simulink model "model_sys"  (R2021a)
settings: Solver=VariableStepAuto  StartTime=0.0  StopTime=100  RelTol=1e-3
values from neighbouring files (symbols this model uses):
  A = [-0.3149 235.8928 0 ... (first row only)    [main.m]    (also in rscale.m = a)
  B = [-5.5079 ... (first row only)    [main.m]    (also in rscale.m = b)
  C = [0 0 1]    [main.m]    (also in rscale.m = c)
  K = lqr(A,B,Q,R)    [main.m]    (also in rscale.m = k)
  N = rscale(A,B,C,D,K)    [main.m]    (also in rscale.m = inv([A,B;C,D])*Z')
undefined symbols (not defined in the file or in its folder): Kf
libraries: simulink x2
settings Model: Creator=artof  LastModifiedBy=artof
settings SolverCC: AlgebraicLoopSolver=TrustRegion
settings DebuggingCC: SFMachineParentedDataDiag=warning

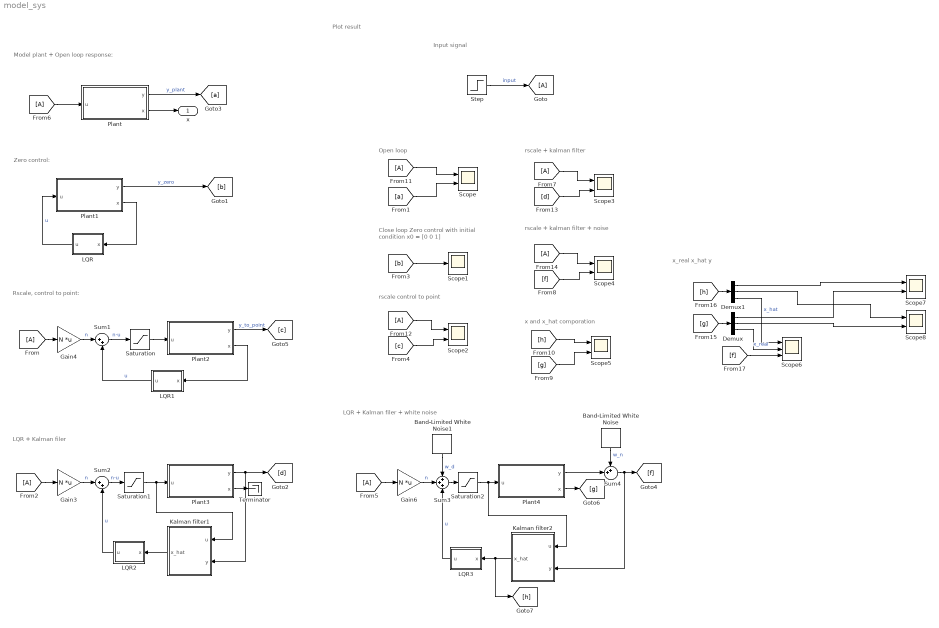
== system model_sys ==
  note: x_real x_hat y
  note: Plot result
  note: Open loop
  note: Input signal
  note: Rscale, control to point:
  note: Zero control:
  note: Model plant + Open loop response:
  note: LQR + Kalman filer
  note: LQR + Kalman filer + white noise
  note: Close loop Zero control with
      | initial condition x0 = [0 0 1]
  note: rscale control to point
  note: rscale + kalman filter
  note: rscale + kalman filter + noise
  note: x and x_hat comporation
  Band-Limited White Noise : simulink/Sources/Band-Limited White Noise  Cov=[0.01]  Ts=0.1  seed=0
  Band-Limited White Noise1 : simulink/Sources/Band-Limited White Noise  Cov=[0.001]  Ts=0.1  seed=0
  Demux : Demux  Outputs=3
  Demux1 : Demux  Outputs=3
  Gain3 : Gain  Gain=N  Multiplication=Matrix(K*u)
  Gain4 : Gain  Gain=N  Multiplication=Matrix(K*u)
  Gain6 : Gain  Gain=N  Multiplication=Matrix(K*u)
  Kalman filter1 : Subsystem
  Kalman filter2 : Subsystem
  LQR : Subsystem
  LQR1 : Subsystem
  LQR2 : Subsystem
  LQR3 : Subsystem
  Plant : Subsystem
  Plant1 : Subsystem
  Plant2 : Subsystem
  Plant3 : Subsystem
  Plant4 : Subsystem
  Saturation : Saturate  UpperLimit=1  LowerLimit=-1
  Saturation1 : Saturate  UpperLimit=1  LowerLimit=-1
  Saturation2 : Saturate  UpperLimit=1  LowerLimit=-1
  Scope{,2..5,7..8} (7 alike) : Scope  NumInputPorts=2
  Scope1 : Scope
  Scope6 : Scope  NumInputPorts=3
  Step : Step  SampleTime=0
  Sum1 : Sum  Inputs=|++
  Sum2 : Sum  Inputs=|++
  Sum3 : Sum  Inputs=+++
  Sum4 : Sum  Inputs=++|
  Terminator : Terminator
  x : Outport
  wires:
  Gain4/1 -> Sum1/1  "n"
  [A] -> Plant/1(u)
  Plant/1(y) -> [a]  "y_plant"
  LQR/1(u) -> Plant1/1(u)  "u"
  Plant/2(x) -> x/1
  Plant1/1(y) -> [b]  "y_zero"
  Plant1/2(x) -> LQR/1(x)
  Plant2/2(x) -> LQR1/1(x)
  LQR1/1(u) -> Sum1/2  "u"
  Gain3/1 -> Sum2/1  "n"
  LQR2/1(u) -> Sum2/2  "u"
  Plant3/1(y) -> [d], Kalman filter1/2(y)
  Sum2/1 -> Saturation1/1  "n-u"
  Gain6/1 -> Sum3/2  "n"
  LQR3/1(u) -> Sum3/3  "u"
  Band-Limited White Noise1/1 -> Sum3/1  "w_d"
  Step/1 -> [A]  "input"
  [a] -> Scope/2
  [A] -> Gain4/1
  Plant2/1(y) -> [c]  "y_to_point"
  [A] -> Gain3/1
  [b] -> Scope1/1
  [c] -> Scope2/2
  [A] -> Gain6/1
  Plant3/2(x) -> Terminator/1
  Kalman filter1/1(x_hat) -> LQR2/1(x)
  Kalman filter2/1(x_hat) -> [h], LQR3/1(x)
  Plant4/1(y) -> Sum4/2
  Plant4/2(x) -> [g]
  Band-Limited White Noise/1 -> Sum4/1  "w_n"
  Sum4/1 -> Kalman filter2/2(y), [f]
  [h] -> Scope5/1
  [g] -> Scope5/2
  [A] -> Scope/1
  [A] -> Scope2/1
  [A] -> Scope3/1
  [d] -> Scope3/2
  [A] -> Scope4/1
  [f] -> Scope4/2
  [g] -> Demux/1
  [h] -> Demux1/1
  Demux1/3 -> Scope6/1  "x_hat"
  Demux/3 -> Scope6/2  "x_real"
  [f] -> Scope6/3
  Sum1/1 -> Saturation/1  "n-u"
  Saturation/1 -> Plant2/1(u)
  Saturation1/1 -> Kalman filter1/1(u), Plant3/1(u)
  Sum3/1 -> Saturation2/1
  Saturation2/1 -> Kalman filter2/1(u), Plant4/1(u)
  Demux1/1 -> Scope7/1
  Demux/1 -> Scope7/2
  Demux1/2 -> Scope8/1
  Demux/2 -> Scope8/2

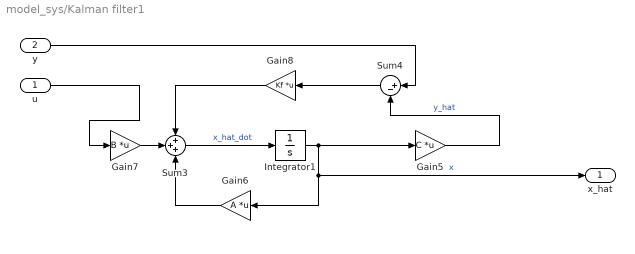
== system model_sys/Kalman filter1 ==
  u : Inport
  y : Inport  Port=2
  Gain5 : Gain  Gain=C  Multiplication=Matrix(K*u)
  Gain6 : Gain  Gain=A  Multiplication=Matrix(K*u)
  Gain7 : Gain  Gain=B  Multiplication=Matrix(K*u)
  Gain8 : Gain  Gain=Kf  Multiplication=Matrix(K*u)
  Integrator1 : Integrator
  Sum3 : Sum  Inputs=+++
  Sum4 : Sum  Inputs=|+-
  x_hat : Outport
  wires:
  Gain5/1 -> Sum4/2  "y_hat"
  Gain6/1 -> Sum3/3
  Gain7/1 -> Sum3/2
  Sum4/1 -> Gain8/1
  Sum3/1 -> Integrator1/1  "x_hat_dot"
  y/1 -> Sum4/1
  Integrator1/1 -> Gain5/1, x_hat/1, Gain6/1  "x"
  Gain8/1 -> Sum3/1
  u/1 -> Gain7/1

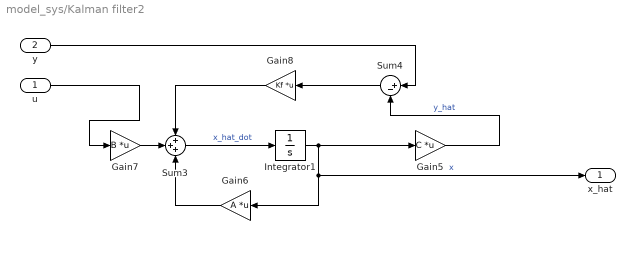
== system model_sys/Kalman filter2 ==
  u : Inport
  y : Inport  Port=2
  Gain5 : Gain  Gain=C  Multiplication=Matrix(K*u)
  Gain6 : Gain  Gain=A  Multiplication=Matrix(K*u)
  Gain7 : Gain  Gain=B  Multiplication=Matrix(K*u)
  Gain8 : Gain  Gain=Kf  Multiplication=Matrix(K*u)
  Integrator1 : Integrator
  Sum3 : Sum  Inputs=+++
  Sum4 : Sum  Inputs=|+-
  x_hat : Outport
  wires:
  Gain5/1 -> Sum4/2  "y_hat"
  Gain6/1 -> Sum3/3
  Gain7/1 -> Sum3/2
  Sum4/1 -> Gain8/1
  Sum3/1 -> Integrator1/1  "x_hat_dot"
  y/1 -> Sum4/1
  Integrator1/1 -> Gain5/1, x_hat/1, Gain6/1  "x"
  Gain8/1 -> Sum3/1
  u/1 -> Gain7/1

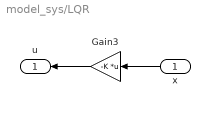
== system model_sys/LQR ==
  x : Inport
  Gain3 : Gain  Gain=-K  Multiplication=Matrix(K*u)
  u : Outport
  wires:
  x/1 -> Gain3/1
  Gain3/1 -> u/1

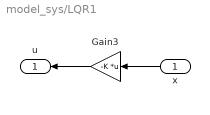
== system model_sys/LQR1 ==
  x : Inport
  Gain3 : Gain  Gain=-K  Multiplication=Matrix(K*u)
  u : Outport
  wires:
  Gain3/1 -> u/1
  x/1 -> Gain3/1

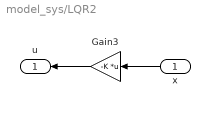
== system model_sys/LQR2 ==
  x : Inport
  Gain3 : Gain  Gain=-K  Multiplication=Matrix(K*u)
  u : Outport
  wires:
  x/1 -> Gain3/1
  Gain3/1 -> u/1

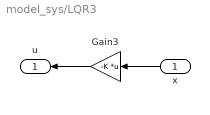
== system model_sys/LQR3 ==
  x : Inport
  Gain3 : Gain  Gain=-K  Multiplication=Matrix(K*u)
  u : Outport
  wires:
  x/1 -> Gain3/1
  Gain3/1 -> u/1

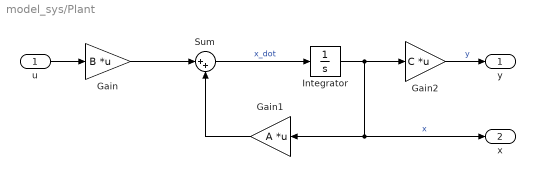
== system model_sys/Plant ==
  u : Inport
  Gain : Gain  Gain=B  Multiplication=Matrix(K*u)
  Gain1 : Gain  Gain=A  Multiplication=Matrix(K*u)
  Gain2 : Gain  Gain=C  Multiplication=Matrix(K*u)
  Integrator : Integrator
  Sum : Sum  Inputs=|++
  y : Outport
  x : Outport  Port=2
  wires:
  Sum/1 -> Integrator/1  "x_dot"
  Gain1/1 -> Sum/2
  Gain2/1 -> y/1  "y"
  Integrator/1 -> Gain2/1, x/1, Gain1/1  "x"
  Gain/1 -> Sum/1
  u/1 -> Gain/1

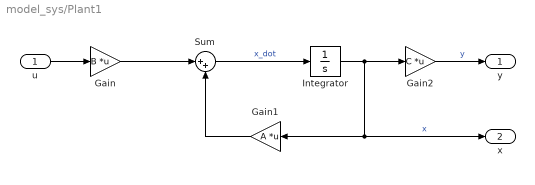
== system model_sys/Plant1 ==
  u : Inport
  Gain : Gain  Gain=B  Multiplication=Matrix(K*u)
  Gain1 : Gain  Gain=A  Multiplication=Matrix(K*u)
  Gain2 : Gain  Gain=C  Multiplication=Matrix(K*u)
  Integrator : Integrator  InitialCondition=[0 0 1]
  Sum : Sum  Inputs=|++
  y : Outport
  x : Outport  Port=2
  wires:
  u/1 -> Gain/1
  Gain/1 -> Sum/1
  Integrator/1 -> Gain1/1, x/1, Gain2/1  "x"
  Gain2/1 -> y/1  "y"
  Gain1/1 -> Sum/2
  Sum/1 -> Integrator/1  "x_dot"

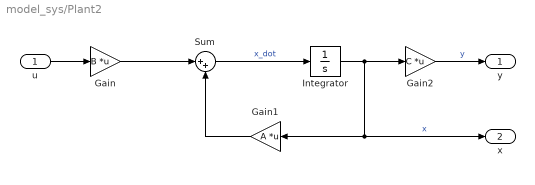
== system model_sys/Plant2 ==
  u : Inport
  Gain : Gain  Gain=B  Multiplication=Matrix(K*u)
  Gain1 : Gain  Gain=A  Multiplication=Matrix(K*u)
  Gain2 : Gain  Gain=C  Multiplication=Matrix(K*u)
  Integrator : Integrator
  Sum : Sum  Inputs=|++
  y : Outport
  x : Outport  Port=2
  wires:
  Sum/1 -> Integrator/1  "x_dot"
  Gain1/1 -> Sum/2
  Gain2/1 -> y/1  "y"
  Integrator/1 -> Gain2/1, x/1, Gain1/1  "x"
  Gain/1 -> Sum/1
  u/1 -> Gain/1

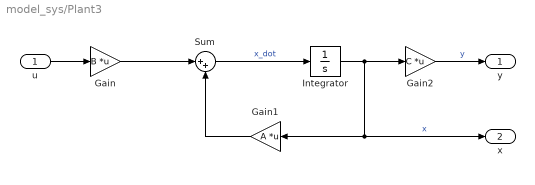
== system model_sys/Plant3 ==
  u : Inport
  Gain : Gain  Gain=B  Multiplication=Matrix(K*u)
  Gain1 : Gain  Gain=A  Multiplication=Matrix(K*u)
  Gain2 : Gain  Gain=C  Multiplication=Matrix(K*u)
  Integrator : Integrator
  Sum : Sum  Inputs=|++
  y : Outport
  x : Outport  Port=2
  wires:
  u/1 -> Gain/1
  Gain/1 -> Sum/1
  Integrator/1 -> Gain1/1, x/1, Gain2/1  "x"
  Gain2/1 -> y/1  "y"
  Gain1/1 -> Sum/2
  Sum/1 -> Integrator/1  "x_dot"

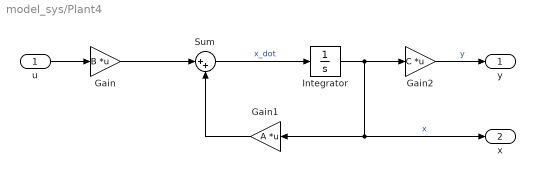
== system model_sys/Plant4 ==
  u : Inport
  Gain : Gain  Gain=B  Multiplication=Matrix(K*u)
  Gain1 : Gain  Gain=A  Multiplication=Matrix(K*u)
  Gain2 : Gain  Gain=C  Multiplication=Matrix(K*u)
  Integrator : Integrator
  Sum : Sum  Inputs=|++
  y : Outport
  x : Outport  Port=2
  wires:
  u/1 -> Gain/1
  Gain/1 -> Sum/1
  Integrator/1 -> Gain1/1, x/1, Gain2/1  "x"
  Gain2/1 -> y/1  "y"
  Gain1/1 -> Sum/2
  Sum/1 -> Integrator/1  "x_dot"
